simulink model "tau_7"  (R2019b)
settings: Solver=VariableStepAuto  StartTime=0.0  StopTime=10  RelTol=1e-3
libraries: simulink x6, slctrlblks x1
settings Model: PacingRate=0.001800  Creator=Sergey  LastModifiedBy=Sergey

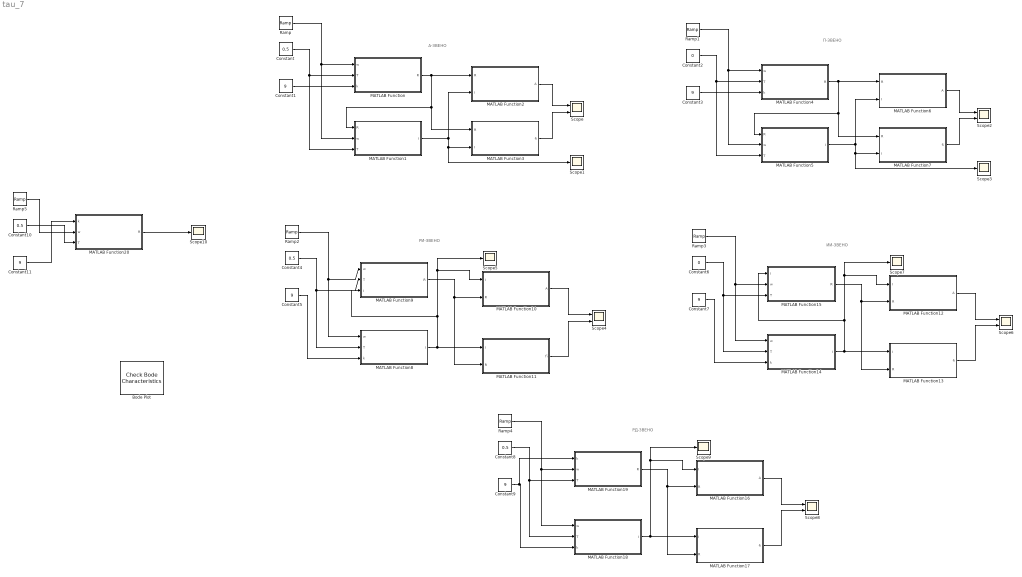
== system tau_7 ==
  note: А-ЗВЕНО
  note: П-ЗВЕНО
  note: РИ-ЗВЕНО
  note: ИИ-ЗВЕНО
  note: РД-ЗВЕНО
  Bode Plot : slctrlblks/Model Verification/Check Bode  Characteristics  InstantiateOnLoad=on  SaveOperatingPoints=off  LinearizationIOs={}  LinearizeAt=SnapshotTimes  SnapshotTimes=[0]  TriggerType=rising  SampleTime=auto  RateConversionMethod=zoh  PreWarpFreq=10  UseExactDelayModel=off  UseFullBlockNameLabels=off  UseBusSignalLabels=off  enabled=on  stopWhenAssertionFail=off  export=off  ViewDlgPos=[1 41 1920 963]  OpenViewOnLoad=off  LaunchViewOnOpen=off  FrequencyUnits=rad/s  MagnitudeUnits=dB  PhaseUnits=deg  TimeUnits=seconds  EnableUpperBound=off  UpperBoundFrequencies=[]  UpperBoundMagnitudes=[]  EnableLowerBound=off  LowerBoundFrequencies=[]  LowerBoundMagnitudes=[]
      settings: SourceProductName=Simulink Control Design
  Constant{,4,8,10} (4 alike) : Constant  Value=0.5
  Constant{1,3,5,7,9,11} (6 alike) : Constant  Value=9
  Constant2 : Constant  Value=0
  Constant6 : Constant  Value=0
  MATLAB Function : MATLAB Function  TreatAsAtomicUnit=on
  MATLAB Function1 : MATLAB Function  TreatAsAtomicUnit=on
  MATLAB Function10 : MATLAB Function  TreatAsAtomicUnit=on
  MATLAB Function11 : MATLAB Function  TreatAsAtomicUnit=on
  MATLAB Function12 : MATLAB Function  TreatAsAtomicUnit=on
  MATLAB Function13 : MATLAB Function  TreatAsAtomicUnit=on
  MATLAB Function14 : MATLAB Function  TreatAsAtomicUnit=on
  MATLAB Function15 : MATLAB Function  TreatAsAtomicUnit=on
  MATLAB Function16 : MATLAB Function  TreatAsAtomicUnit=on
  MATLAB Function17 : MATLAB Function  TreatAsAtomicUnit=on
  MATLAB Function18 : MATLAB Function  TreatAsAtomicUnit=on
  MATLAB Function19 : MATLAB Function  TreatAsAtomicUnit=on
  MATLAB Function2 : MATLAB Function  TreatAsAtomicUnit=on
  MATLAB Function20 : MATLAB Function  TreatAsAtomicUnit=on
  MATLAB Function3 : MATLAB Function  TreatAsAtomicUnit=on
  MATLAB Function4 : MATLAB Function  TreatAsAtomicUnit=on
  MATLAB Function5 : MATLAB Function  TreatAsAtomicUnit=on
  MATLAB Function6 : MATLAB Function  TreatAsAtomicUnit=on
  MATLAB Function7 : MATLAB Function  TreatAsAtomicUnit=on
  MATLAB Function8 : MATLAB Function  TreatAsAtomicUnit=on
  MATLAB Function9 : MATLAB Function  TreatAsAtomicUnit=on
  Ramp{,1..4} (5 alike) : simulink/Sources/Ramp  slope=1  start=0  InitialOutput=0
  Ramp5 : simulink/Sources/Ramp  slope=.0001  start=0  InitialOutput=0
  Scope{,2,4,6,8} (5 alike) : Scope  NumInputPorts=2
  Scope{1,3,5,7,9..10} (6 alike) : Scope
  wires:
  Ramp/1 -> MATLAB Function1/2(w), MATLAB Function/1(w)
  Constant/1 -> MATLAB Function1/3(T), MATLAB Function/2(T)
  Constant1/1 -> MATLAB Function/3(k)
  MATLAB Function/1(R) -> MATLAB Function3/1(R), MATLAB Function1/1(R), MATLAB Function2/1(R)
  MATLAB Function1/1(I) -> Scope1/1, MATLAB Function3/2(I), MATLAB Function2/2(I)
  MATLAB Function2/1(A) -> Scope/1
  MATLAB Function3/1(fi) -> Scope/2
  MATLAB Function7/1(fi) -> Scope2/2
  MATLAB Function6/1(A) -> Scope2/1
  MATLAB Function5/1(I) -> MATLAB Function6/2(I), MATLAB Function7/2(I), Scope3/1
  MATLAB Function4/1(R) -> MATLAB Function6/1(R), MATLAB Function5/1(R), MATLAB Function7/1(R)
  Constant3/1 -> MATLAB Function4/3(k)
  Constant2/1 -> MATLAB Function4/2(T), MATLAB Function5/3(T)
  Ramp1/1 -> MATLAB Function4/1(w), MATLAB Function5/2(w)
  MATLAB Function11/1(fi) -> Scope4/2
  MATLAB Function10/1(A) -> Scope4/1
  MATLAB Function9/1(R) -> MATLAB Function11/2(R), MATLAB Function10/2(R)
  MATLAB Function8/1(I) -> Scope5/1, MATLAB Function10/1(I), MATLAB Function9/3(I), MATLAB Function11/1(I)
  Constant5/1 -> MATLAB Function8/3(k)
  Constant4/1 -> MATLAB Function8/2(T), MATLAB Function9/2(T)
  Ramp2/1 -> MATLAB Function8/1(w), MATLAB Function9/1(w)
  Ramp3/1 -> MATLAB Function15/2(w), MATLAB Function14/1(w)
  Constant6/1 -> MATLAB Function15/3(T), MATLAB Function14/2(T)
  Constant7/1 -> MATLAB Function14/3(k)
  MATLAB Function14/1(I) -> MATLAB Function13/1(I), MATLAB Function15/1(I), MATLAB Function12/1(I), Scope7/1
  MATLAB Function15/1(R) -> MATLAB Function12/2(R), MATLAB Function13/2(R)
  MATLAB Function12/1(A) -> Scope6/1
  MATLAB Function13/1(fi) -> Scope6/2
  Ramp4/1 -> MATLAB Function19/2(w), MATLAB Function18/1(w)
  Constant8/1 -> MATLAB Function19/3(T), MATLAB Function18/2(T)
  Constant9/1 -> MATLAB Function19/1(k), MATLAB Function18/3(k)
  MATLAB Function18/1(I) -> MATLAB Function17/1(I), MATLAB Function16/1(I), Scope9/1
  MATLAB Function19/1(R) -> MATLAB Function16/2(R), MATLAB Function17/2(R)
  MATLAB Function16/1(A) -> Scope8/1
  MATLAB Function17/1(fi) -> Scope8/2
  Constant11/1 -> MATLAB Function20/1(k)
  Constant10/1 -> MATLAB Function20/3(T)
  MATLAB Function20/1(R) -> Scope10/1
  Ramp5/1 -> MATLAB Function20/2(w)

== matlab function tau_7/MATLAB Function1 ==
  data: R input; w input; I output; T input
function I = fcn(R,w,T)

I = R*w*T;
I = -I;

== matlab function tau_7/MATLAB Function ==
  data: w input; R output; T input; k input
function R = fcn(w,T,k)

R = k/(1+w^2*T^2);

== matlab function tau_7/MATLAB Function2 ==
  data: R input; I input; A output
function A = fcn(R,I)

A = R^2+I^2;
A = sqrt(A);

== matlab function tau_7/MATLAB Function3 ==
  data: R input; I input; fi output
function fi = fcn(R,I)


fi = atan2(I,R);

== matlab function tau_7/MATLAB Function4 ==
  data: w input; R output; T input; k input
function R = fcn(w,T,k)

R = k/(1+w^2*T^2);

== matlab function tau_7/MATLAB Function5 ==
  data: R input; w input; I output; T input
function I = fcn(R,w,T)

I = R*w*T;
I = -I;

== matlab function tau_7/MATLAB Function6 ==
  data: R input; I input; A output
function A = fcn(R,I)

A = R^2+I^2;
A = sqrt(A);

== matlab function tau_7/MATLAB Function7 ==
  data: R input; I input; fi output
function fi = fcn(R,I)


fi = atan2(I,R);

== matlab function tau_7/MATLAB Function10 ==
  data: I input; R input; A output
function A = fcn(I,R)

A = R^2+I^2;
A = sqrt(A);

== matlab function tau_7/MATLAB Function11 ==
  data: I input; R input; fi output
function fi = fcn(I,R)


fi = atan2(I,R);

== matlab function tau_7/MATLAB Function8 ==
  data: w input; I output; T input; k input
function I = fcn(w,T,k)

I = k/(w*(1+w^2*T^2));
I = -I;

== matlab function tau_7/MATLAB Function9 ==
  data: w input; T input; I input; R output
function R = fcn(w,T,I)


R = I*w*T;

== matlab function tau_7/MATLAB Function12 ==
  data: I input; R input; A output
function A = fcn(I,R)

A = R^2+I^2;
A = sqrt(A);

== matlab function tau_7/MATLAB Function13 ==
  data: I input; R input; fi output
function fi = fcn(I,R)


fi = atan2(I,R);

== matlab function tau_7/MATLAB Function14 ==
  data: w input; I output; T input; k input
function I = fcn(w,T,k)

I = k/(w*(1+w^2*T^2));
I = -I;

== matlab function tau_7/MATLAB Function15 ==
  data: I input; w input; R output; T input
function R = fcn(I,w,T)


R = I*w*T;

== matlab function tau_7/MATLAB Function16 ==
  data: I input; R input; A output
function A = fcn(I,R)

A = R^2+I^2;
A = sqrt(A);

== matlab function tau_7/MATLAB Function17 ==
  data: I input; R input; fi output
function fi = fcn(I,R)


fi = atan2(I,R);

== matlab function tau_7/MATLAB Function18 ==
  data: w input; I output; T input; k input
function I = fcn(w,T,k)

I = (k*w)/(1+w^2*T^2);

== matlab function tau_7/MATLAB Function19 ==
  data: k input; w input; R output; T input
function R = fcn(k,w,T)


R = (w^2*T*k)/(1+w^2*T^2);

== matlab function tau_7/MATLAB Function20 ==
  data: k input; w input; T input; R output
function R = fcn(k,w,T)


R = k/(w*sqrt(1+w^2*T^2));
